simulink model "cascaded_system"  (Simulink 6.0)
settings: Solver=ode45  StartTime=0.0  StopTime=10  RelTol=1e-3
undefined symbols (not defined in the file or in its folder): Fs, read, rfdata
libraries: rfports1 x8, rftxlines1 x6, rfamplifiers1 x4, dspsnks4 x1, simulink x1, dspsrcs4 x1
settings Model: Creator=RobertZ  LastModifiedBy=rzeng  ProdHWDeviceType=Specified
settings DataIOCC: SaveOutput=off  SaveTime=off  SignalLoggingName=sigsOut
settings DebuggingCC: CheckExecutionContextPreStartOutputMsg=on  CheckExecutionContextRuntimeOutputMsg=on  SolverPrmCheckMsg=none
settings HardwareCC: ProdHWDeviceType=Specified
settings ModelReferenceCC: UpdateModelReferenceTargets=IfOutOfDate
settings SFSimCC: SFSimApplyToAllLibs=on  SFSimBuildMode=Incremental

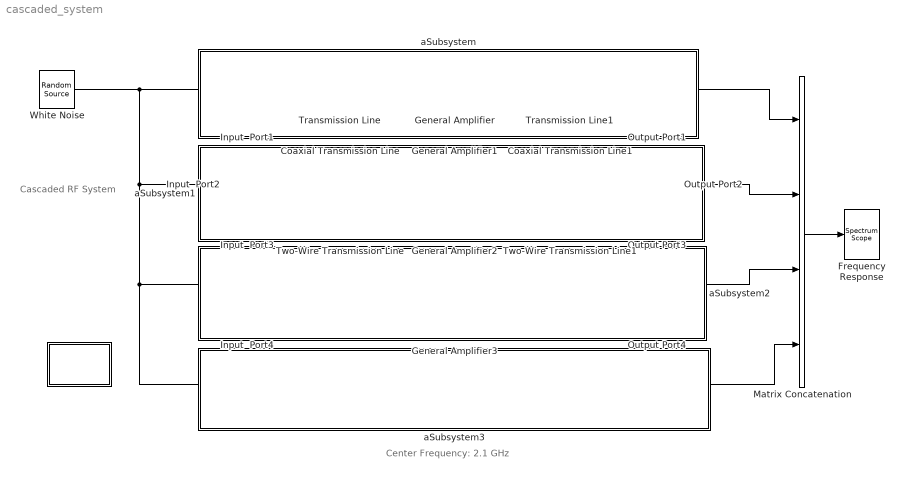
== system cascaded_system ==
  note: Cascaded
      | RF System
  note: Center Frequency: 2.1 GHz
  " " : Subsystem  PropExecContextAcrossSSBoundary=on
      mask Type: Interpolation filter info block
      mask Display: disp('Info')
  Coaxial Transmission Line : rftxlines1/Coaxial Transmission Line  PhysicalDomain=rfsystemsdomain  SubClassName=coaxial  LeftPortType=p1  RightPortType=p1  LConnTagsString=__newl0  RConnTagsString=__newr0  OuterRadius=5e-3  InnerRadius=1.411e-3  MuR=1  EpsilonR=2.3  SigmaCond=6.55e7  SigmaDiel=0  LineLength=1  StubMode=Not a stub  Termination=Open  DisplayData=off  PlotFreq=Derived from Input Port parameters  PlotFreqNoSim=User specified  Freq=[1.85e9:1e8:2.35e9]  AllPlotType=X-Y plane  NetworkData=S21  SmithData=S11  PolarData=S11  ComplexFormat=Magnitude (decibels)  DBFormat=Magnitude (decibels)  NoneFormat=None
  Coaxial Transmission Line1 : rftxlines1/Coaxial Transmission Line  PhysicalDomain=rfsystemsdomain  SubClassName=coaxial  LeftPortType=p1  RightPortType=p1  LConnTagsString=__newl0  RConnTagsString=__newr0  OuterRadius=5e-3  InnerRadius=1.411e-3  MuR=1  EpsilonR=2.3  SigmaCond=6.55e7  SigmaDiel=0  LineLength=1  StubMode=Not a stub  Termination=Open  DisplayData=off  PlotFreq=Derived from Input Port parameters  PlotFreqNoSim=User specified  Freq=[1.85e9:1e8:2.35e9]  AllPlotType=X-Y plane  NetworkData=S21  SmithData=S11  PolarData=S11  ComplexFormat=Magnitude (decibels)  DBFormat=Magnitude (decibels)  NoneFormat=None
  Frequency Response : dspsnks4/Spectrum Scope  ScopeProperties=off  Domain=Frequency  HorizSpan=1  UseBuffer=on  BufferSize=1024  Overlap=512  inpFftLenInherit=on  FFTlength=1024  numAvg=100  DisplayProperties=off  AxisGrid=on  Memory=off  FrameNumber=on  AxisLegend=on  AxisZoom=off  OpenScopeAtSimStart=on  OpenScopeImmediately=off  FigPos=[271 297 418 259]  AxisProperties=off  XUnits=Hertz  XRange=[-Fs/2...Fs/2]  InheritXIncr=on  XIncr=1.0  XLabel=Samples  YUnits=dB  YLabel=Magnitude, dB  LineProperties=on  LineStyles=--  LineColors=|[1 0 0]|[0 1 0]|[0 0 1]
      settings: YMin=-12.2966964567787  YMax=16.6066750307094
  General Amplifier{,1..3} (4 alike) : rfamplifiers1/General Amplifier  PhysicalDomain=rfsystemsdomain  SubClassName=general-amplifier  LeftPortType=p1  RightPortType=p1  LConnTagsString=__newl0  RConnTagsString=__newr0  RFDATA=read(rfdata.data, 'default.s2p')  InterpMethod=Linear  IP3Type=OIP3  IIP3=inf  OIP3=inf  NF=0  DisplayData=off  PlotFreq=Derived from Input Port parameters  PlotFreqNoSim=Extracted from RFDATA object  Freq=[1e9:1e8:2.9e9]  AllPlotType=X-Y plane  NetworkData=S21  PowerData=S11  SmithData=S11  PolarData=S11  ComplexFormat=Magnitude (decibels)  DBFormat=Magnitude (decibels)  PowerFormat=dBm  PhaseFormat=Angle (degrees)  NoneFormat=None
  Input  Port1 : rfports1/Input Port  Description=source block  MaxLength=128  Fc=2.1e9  Ts=2e-9  Zs=50  NoiseFlag=off  seed=67987  GoToTag=BBACKMAKRNOADGRSSILVGMW
  Input  Port2 : rfports1/Input Port  Description=source block  MaxLength=128  Fc=2.1e9  Ts=2e-9  Zs=50  NoiseFlag=off  seed=67987  GoToTag=ACBDAABLSOPBEHSTTJMWHNX
  Input  Port3 : rfports1/Input Port  Description=source block  MaxLength=128  Fc=2.1e9  Ts=2e-9  Zs=50  NoiseFlag=off  seed=67987  GoToTag=BACEBBCMTPQCFITUUKNXIOY
  Input  Port4 : rfports1/Input Port  Description=source block  MaxLength=128  Fc=2.1e9  Ts=2e-9  Zs=50  NoiseFlag=off  seed=67987  GoToTag=ABDFCCDNUQRDGJUVVLOYJPZ
  Matrix Concatenation : simulink/Math Operations/Matrix Concatenation  numInports=4  catMethod=Horizontal
  Output Port1 : rfports1/Output Port  Zl=50  num_Models=1  GoToTag=BBACKMAKRNOADGRSSILVGMW  DisplayData=off  PlotFreq=Derived from Input Port parameters  Freq=1e9:1e8:3e9  AllPlotType=Composite data  NoBudgetPlot=Composite data  NetworkData=S11  SmithData=S11  PolarData=S11  ComplexFormat=Magnitude (decibels)  DBFormat=Magnitude (decibels)  DBMFormat=dBm  NoneFormat=None
  Output Port2 : rfports1/Output Port  Zl=50  num_Models=1  GoToTag=ACBDAABLSOPBEHSTTJMWHNX  DisplayData=off  PlotFreq=Derived from Input Port parameters  Freq=1e9:1e8:3e9  AllPlotType=Composite data  NoBudgetPlot=Composite data  NetworkData=S11  SmithData=S11  PolarData=S11  ComplexFormat=Magnitude (decibels)  DBFormat=Magnitude (decibels)  DBMFormat=dBm  NoneFormat=None
  Output Port3 : rfports1/Output Port  Zl=50  num_Models=1  GoToTag=BACEBBCMTPQCFITUUKNXIOY  DisplayData=off  PlotFreq=Derived from Input Port parameters  Freq=1e9:1e8:3e9  AllPlotType=Composite data  NoBudgetPlot=Composite data  NetworkData=S11  SmithData=S11  PolarData=S11  ComplexFormat=Magnitude (decibels)  DBFormat=Magnitude (decibels)  DBMFormat=dBm  NoneFormat=None
  Output Port4 : rfports1/Output Port  Zl=50  num_Models=1  GoToTag=ABDFCCDNUQRDGJUVVLOYJPZ  DisplayData=off  PlotFreq=Derived from Input Port parameters  Freq=1e9:1e8:3e9  AllPlotType=Composite data  NoBudgetPlot=Composite data  NetworkData=S11  SmithData=S11  PolarData=S11  ComplexFormat=Magnitude (decibels)  DBFormat=Magnitude (decibels)  DBMFormat=dBm  NoneFormat=None
  Transmission Line : rftxlines1/Transmission Line  PhysicalDomain=rfsystemsdomain  SubClassName=txline  LeftPortType=p1  RightPortType=p1  LConnTagsString=__newl0  RConnTagsString=__newr0  Z0=50  PV=299792458  Loss=5  LineLength=1  StubMode=Not a stub  Termination=Open  DisplayData=off  PlotFreq=Derived from Input Port parameters  PlotFreqNoSim=User specified  Freq=[1.85e9:1e8:2.35e9]  AllPlotType=X-Y plane  NetworkData=S21  SmithData=S11  PolarData=S11  ComplexFormat=Magnitude (decibels)  DBFormat=Magnitude (decibels)  NoneFormat=None
  Transmission Line1 : rftxlines1/Transmission Line  PhysicalDomain=rfsystemsdomain  SubClassName=txline  LeftPortType=p1  RightPortType=p1  LConnTagsString=__newl0  RConnTagsString=__newr0  Z0=50  PV=299792458  Loss=5  LineLength=1  StubMode=Not a stub  Termination=Open  DisplayData=off  PlotFreq=Derived from Input Port parameters  PlotFreqNoSim=User specified  Freq=[1.85e9:1e8:2.35e9]  AllPlotType=X-Y plane  NetworkData=S12  SmithData=S11  PolarData=S11  ComplexFormat=Magnitude (decibels)  DBFormat=Magnitude (decibels)  NoneFormat=None
  Two-Wire Transmission Line : rftxlines1/Two-Wire Transmission Line  PhysicalDomain=rfsystemsdomain  SubClassName=twowire  LeftPortType=p1  RightPortType=p1  LConnTagsString=__newl0  RConnTagsString=__newr0  Radius=2.0574e-3  Separation=4.966e-3  MuR=1  EpsilonR=2.3  SigmaCond=6.55e6  SigmaDiel=0.002  LineLength=1  StubMode=Not a stub  Termination=Open  DisplayData=off  PlotFreq=Derived from Input Port parameters  PlotFreqNoSim=User specified  Freq=1.85e9:1e8:2.35e9  AllPlotType=X-Y plane  NetworkData=S21  SmithData=S11  PolarData=S11  ComplexFormat=Magnitude (decibels)  DBFormat=Magnitude (decibels)  NoneFormat=None
  Two-Wire Transmission Line1 : rftxlines1/Two-Wire Transmission Line  PhysicalDomain=rfsystemsdomain  SubClassName=twowire  LeftPortType=p1  RightPortType=p1  LConnTagsString=__newl0  RConnTagsString=__newr0  Radius=2.0574e-3  Separation=4.966e-3  MuR=1  EpsilonR=2.3  SigmaCond=6.55e6  SigmaDiel=0.002  LineLength=1  StubMode=Not a stub  Termination=Open  DisplayData=off  PlotFreq=Derived from Input Port parameters  PlotFreqNoSim=User specified  Freq=1.85e9:1e8:2.35e9  AllPlotType=X-Y plane  NetworkData=S21  SmithData=S11  PolarData=S11  ComplexFormat=Magnitude (decibels)  DBFormat=Magnitude (decibels)  NoneFormat=None
  White Noise : dspsrcs4/Random Source  SrcType=Gaussian  NormMethod=Ziggurat  CltLength=12  Min=-1  Max=1  Mean=0  Var=1  RepMode=Not repeatable  rawSeed=1  Inherit=off  SampMode=Discrete  SampTime=2e-9  SampFrame=256  DataType=Double  OutComplex=Complex
  aSubsystem : Subsystem  PropExecContextAcrossSSBoundary=on
      mask Display: disp('')
  aSubsystem1 : Subsystem  PropExecContextAcrossSSBoundary=on
      mask Display: disp('')
  aSubsystem2 : Subsystem  PropExecContextAcrossSSBoundary=on
      mask Display: disp('')
  aSubsystem3 : Subsystem  PropExecContextAcrossSSBoundary=on
      mask Display: disp('')
  wires:
  White Noise/1 -> Input  Port4/1, Input  Port3/1, Input  Port2/1, Input  Port1/1
  Matrix Concatenation/1 -> Frequency Response/1
  Output Port1/1 -> Matrix Concatenation/1
  Output Port2/1 -> Matrix Concatenation/2
  Output Port3/1 -> Matrix Concatenation/3
  Output Port4/1 -> Matrix Concatenation/4
  connections:
  Transmission Line1/RConn1 -- Output Port1/LConn1
  General Amplifier/RConn1 -- Transmission Line1/LConn1
  Input  Port1/RConn1 -- Transmission Line/LConn1
  Transmission Line/RConn1 -- General Amplifier/LConn1
  Coaxial Transmission Line1/RConn1 -- Output Port2/LConn1
  General Amplifier1/RConn1 -- Coaxial Transmission Line1/LConn1
  Input  Port2/RConn1 -- Coaxial Transmission Line/LConn1
  Coaxial Transmission Line/RConn1 -- General Amplifier1/LConn1
  Two-Wire Transmission Line1/RConn1 -- Output Port3/LConn1
  General Amplifier2/RConn1 -- Two-Wire Transmission Line1/LConn1
  Input  Port3/RConn1 -- Two-Wire Transmission Line/LConn1
  Two-Wire Transmission Line/RConn1 -- General Amplifier2/LConn1
  General Amplifier3/RConn1 -- Output Port4/LConn1
  Input  Port4/RConn1 -- General Amplifier3/LConn1

== system cascaded_system/  ==
  note: Cascaded RF System
      |
      | This demo shows how to cascade blocks from RF Physical Library.
      | In each of the first three yellow diagrams from the top,
      | three physical blocks are cascaded:
      | Different types of transmission lines are used in the diagrams
      | and they have different loss. However,
      | their characteristic impedances are all approximately 50 Ohm.
      |
      | The spectrum plot shows frequency ranging from
      | 1.85GHz to 2.35GHz centered at 2.1GHz.
      |
      | If you want to see the frequency response centered at other RF frequency,
      | you need to change the Center frequency parameter in the
      | 'Input Port' block.
      |
      | If you want to change the range of frequency response that is determined by
      | the Sample time parameter specified in the 'Input Port' and 'White Noise' blocks,
      | you need to change the Sample time parameter in both blocks.

== system cascaded_system/aSubsystem ==

== system cascaded_system/aSubsystem1 ==

== system cascaded_system/aSubsystem2 ==

== system cascaded_system/aSubsystem3 ==
